simulink model "reward202510141003"  (R2025a)
settings: Solver=VariableStepAuto  StartTime=0.0  StopTime=10.0  RelTol=1e-3
libraries: fuzblock x2
settings Model: Creator=86138  LastModifiedBy=86138

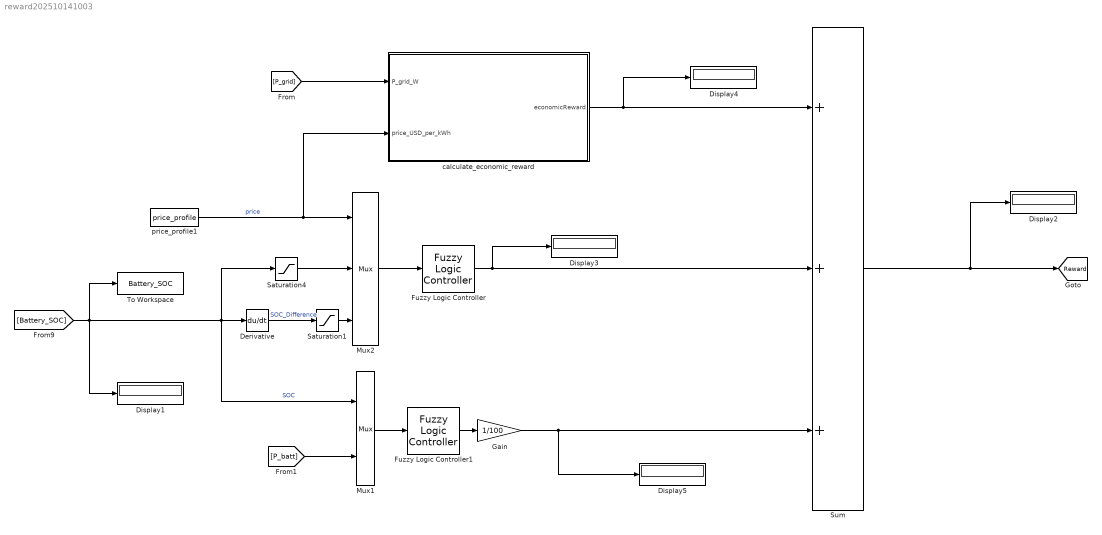
== system reward202510141003 ==
  Derivative : Derivative
  Display{1..5} (5 alike) : Display
  Fuzzy Logic Controller : fuzblock/Fuzzy Logic  Controller  FIS='Battery_State_Type2.fis'  OutputSampleNumber=101  DataType=double  UseLookupTable=off  NumBreakpoints=10  FuzzifiedInputs=off  RuleFiringStrengths=off  RuleOutputs=off  AggregatedOutputs=off  SimulateUsing=Interpreted execution  OutOfRangeInputValueMessage=warning  NoRuleFiredMessage=warning  EmptyOutputFuzzySetMessage=warning
  Fuzzy Logic Controller1 : fuzblock/Fuzzy Logic  Controller  FIS='SOCProtector_Type2.fis'  OutputSampleNumber=101  DataType=double  UseLookupTable=off  NumBreakpoints=10  FuzzifiedInputs=off  RuleFiringStrengths=off  RuleOutputs=off  AggregatedOutputs=off  SimulateUsing=Interpreted execution  OutOfRangeInputValueMessage=warning  NoRuleFiredMessage=warning  EmptyOutputFuzzySetMessage=warning
  Gain : Gain  Gain=1/100
  Mux1 : Mux  Inputs=2
  Mux2 : Mux  Inputs=3
  Saturation1 : Saturate  UpperLimit=100  LowerLimit=-100  LinearizeAsGain=off  ZeroCross=off  OutMin=-100  RndMeth=Simplest
  Saturation4 : Saturate  UpperLimit=100  LowerLimit=0  LinearizeAsGain=off  ZeroCross=off  OutMin=0  RndMeth=Simplest
  Sum : Sum  Inputs=+++
  To Workspace : ToWorkspace  VariableName=Battery_SOC  SampleTime=3600
      settings: Save2DSignal=2-D array (concatenate along first dimension)
  calculate_economic_reward : MATLAB Function  TreatAsAtomicUnit=on
  price_profile1 : FromWorkspace  VariableName=price_profile
  tag scope: Reward=global
  wires:
  Derivative/1 -> Saturation1/1  "SOC_Difference"
  Sum/1 -> Display2/1, [Reward]
  [P_batt] -> Mux1/2
  price_profile1/1 -> calculate_economic_reward/2(price_USD_per_kWh), Mux2/1  "price"
  Saturation1/1 -> Mux2/3
  [P_grid] -> calculate_economic_reward/1(P_grid_W)
  calculate_economic_reward/1(economicReward) -> Sum/1, Display4/1
  Mux2/1 -> Fuzzy Logic Controller/1
  Fuzzy Logic Controller1/1 -> Gain/1
  Saturation4/1 -> Mux2/2
  [Battery_SOC] -> Display1/1, To Workspace/1, Derivative/1, Mux1/1, Saturation4/1  "SOC"
  Fuzzy Logic Controller/1 -> Display3/1, Sum/2
  Mux1/1 -> Fuzzy Logic Controller1/1
  Gain/1 -> Display5/1, Sum/3

== matlab function reward202510141003/calculate_economic_reward ==
  data: P_grid_W input; economicReward output; price_USD_per_kWh input
function economicReward = calculate_economic_reward(P_grid_W, price_USD_per_kWh)
%CALCULATE_ECONOMIC_REWARD Compute the economic reward component.
%   economicReward = CALCULATE_ECONOMIC_REWARD(P_grid_W, price_USD_per_kWh)
%   returns the reward associated with buying or selling power at the
%   current price. Positive values represent revenue, negative values
%   represent cost. Internal constants determine penalty strength.
%
%   Inputs:
%       P_grid_W          - Grid exchange power [W], >0 buy, <0 sell.
%       price_USD_per_kWh - Real-time energy price [$/kWh].
%
%   Output:
%       economicReward    - Scalar economic reward contribution.

    arguments
        P_grid_W (1,1) double
        price_USD_per_kWh (1,1) double
    end

    % Tunable constants (adjust in code if needed).
    peakPowerThresholdW = 15e3;  % [W] Peak import threshold.
    highPriceThreshold = 0.40;   % [$/kWh] High price definition.
    penaltyFactor = 5e-8;        % Quadratic penalty scale.
    timeStepHours = 1.0;         % Simulation step duration [h].

    % Core transaction term: revenue when exporting, cost when importing.
    P_grid_kW = P_grid_W / 1000.0;
    linear_reward = -(P_grid_kW * price_USD_per_kWh * timeStepHours);

    % Peak power penalty discourages expensive peak-hour imports.
    peak_penalty = 0.0;
    if (P_grid_W > 0) && (P_grid_W > peakPowerThresholdW) && (price_USD_per_kWh > highPriceThreshold)
        peak_penalty = -penaltyFactor * (P_grid_W ^ 2);
    end

    economicReward = linear_reward + peak_penalty;
end
